simulink model "inverter_base"  (R2024a)
settings: Solver=VariableStepAuto  StartTime=0.0  StopTime=0.5  RelTol=1e-3
undefined symbols (not defined in the file): C_filter, L1, L2, R_damp, R_series1, R_series2
libraries: spsSeriesRLCBranchLib x5, spsIGBTDiodeLib x4, spsVoltageMeasurementLib x4, spsCurrentMeasurementLib x3, spsDCVoltageSourceLib x1, spspowerguiLib x1
settings Model: Creator=user  LastModifiedBy=user

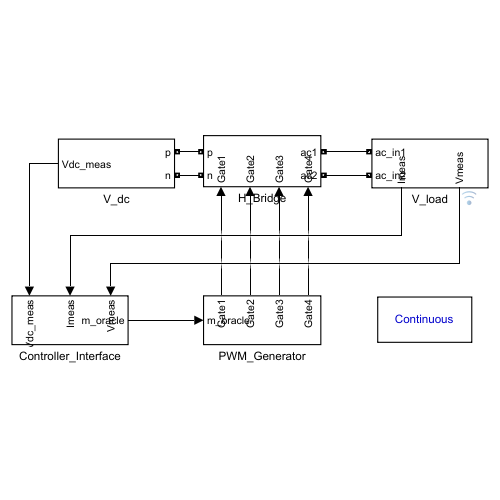
[thumbnail: Simulink's stored preview of the top-level diagram]
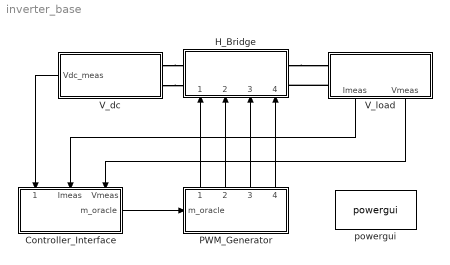
== system inverter_base ==
  Controller_Interface : Subsystem
      settings: PortSchema="{\"entries\":[{\"content\":{\"sides\":[{\"content\":{},\"type\":\"ConnectorPlacement.EquallySpacedRectSide\",\"uuid\":\"9a16cef6-3ad2-4b7e-9cb0-1cc099279abc\"},{\"content\":{\"connectorIds\":[\"Out1\"],\"side\":\"RIGHT\"},\"type\":\"ConnectorPlacement.EquallySpacedRectSide\",\"uuid\":\"1641ad69-610c-4562-8ab1-2b7cab01bb45\"},{\"content\":{\"connectorIds\":[\"In1\",\"In2\",\"In3\"],\"side\":\"TOP\"},\"type\":\"ConnectorPlacement.EquallySpacedRectSide\",\"uuid\":\"2c8d616f-a4b3-4b7e-a4a8-8a8252d3766c\"}]},\"type\":\"ConnectorPlacement.EquallySpacedConnector\",\"uuid\":\"2c20ff8a-19ba-4bf3-9a10-031d18a0fe42\"}],\"packageUris\":[\"http://schema.mathworks.com/mf0/Connector/R2020b\"],\"version\":\"1.0\"}"
  H_Bridge : Subsystem
      settings: PortSchema="{\"entries\":[{\"content\":{\"sides\":[{\"content\":{\"connectorIds\":[\"LConn1\",\"LConn2\"]},\"type\":\"ConnectorPlacement.EquallySpacedRectSide\",\"uuid\":\"86489d03-198d-4d40-a5a9-bb389f882c52\"},{\"content\":{\"connectorIds\":[\"RConn1\",\"RConn2\"],\"side\":\"RIGHT\"},\"type\":\"ConnectorPlacement.EquallySpacedRectSide\",\"uuid\":\"3ab0f84a-d55a-4cb1-90b5-b7bc956b0bff\"},{\"content\":{\"side\":\"TOP\"},\"type\":\"ConnectorPlacement.EquallySpacedRectSide\",\"uuid\":\"23383f72-5c44-4878-8c70-727696e5b54e\"},{\"content\":{\"connectorIds\":[\"In1\",\"In2\",\"In3\",\"In4\"],\"side\":\"BOTTOM\"},\"type\":\"ConnectorPlacement.EquallySpacedRectSide\",\"uuid\":\"2d41232e-3b94-4b8d-8bb1-4fff68b55e28\"}]},\"type\":\"ConnectorPlacement.EquallySpacedConnector\",\"uuid\":\"d39d40f2-549c-43a5-af7d-108fa7f92b85\"}],\"packageUris\":[\"http://schema.mathworks.com/mf0/Connector/R2020b\"],\"version\":\"1.0\"}"
  PWM_Generator : Subsystem
      settings: PortSchema="{\"entries\":[{\"content\":{\"sides\":[{\"content\":{\"connectorIds\":[\"In1\"]},\"type\":\"ConnectorPlacement.EquallySpacedRectSide\",\"uuid\":\"400e631f-5393-4580-84ff-cf0e7a5cd70f\"},{\"content\":{\"side\":\"RIGHT\"},\"type\":\"ConnectorPlacement.EquallySpacedRectSide\",\"uuid\":\"fe659c7d-79b6-4ef2-8759-c3fa799506d4\"},{\"content\":{\"connectorIds\":[\"Out1\",\"Out2\",\"Out3\",\"Out4\"],\"side\":\"TOP\"},\"type\":\"ConnectorPlacement.EquallySpacedRectSide\",\"uuid\":\"3e9a409d-18be-4b1d-9bb1-0d4655d86115\"}]},\"type\":\"ConnectorPlacement.EquallySpacedConnector\",\"uuid\":\"2db352b5-5690-44f0-aaa9-f258dc14ff92\"}],\"packageUris\":[\"http://schema.mathworks.com/mf0/Connector/R2020b\"],\"version\":\"1.0\"}"
  V_dc : Subsystem
      settings: PortSchema="{\"entries\":[{\"content\":{\"sides\":[{\"content\":{\"connectorIds\":[\"Out1\"]},\"type\":\"ConnectorPlacement.EquallySpacedRectSide\",\"uuid\":\"2cb68214-b015-46eb-8931-ac971d781749\"},{\"content\":{\"connectorIds\":[\"RConn1\",\"RConn2\"],\"side\":\"RIGHT\"},\"type\":\"ConnectorPlacement.EquallySpacedRectSide\",\"uuid\":\"9d50e4c1-4d5c-4242-a631-3bd3e824d3e8\"},{\"content\":{\"side\":\"TOP\"},\"type\":\"ConnectorPlacement.EquallySpacedRectSide\",\"uuid\":\"afad02bd-f500-4aa5-b819-b29c92a1000c\"},{\"content\":{\"side\":\"BOTTOM\"},\"type\":\"ConnectorPlacement.EquallySpacedRectSide\",\"uuid\":\"d1fcf53c-bcc4-4453-a05d-028d0bdae388\"}]},\"type\":\"ConnectorPlacement.EquallySpacedConnector\",\"uuid\":\"cb259193-6dd3-4248-8ce6-c0a2b09c3017\"}],\"packageUris\":[\"http://schema.mathworks.com/mf0/Connector/R2020b\"],\"version\":\"1.0\"}"
  V_load : Subsystem
      settings: PortSchema="{\"entries\":[{\"content\":{\"sides\":[{\"content\":{\"connectorIds\":[\"LConn1\",\"LConn2\"]},\"type\":\"ConnectorPlacement.EquallySpacedRectSide\",\"uuid\":\"e1621729-e0e3-4406-9722-79cabe3ad09b\"},{\"content\":{\"side\":\"RIGHT\"},\"type\":\"ConnectorPlacement.EquallySpacedRectSide\",\"uuid\":\"78182f87-e3d0-42da-9ed2-9ba8ffc9d138\"},{\"content\":{\"side\":\"TOP\"},\"type\":\"ConnectorPlacement.EquallySpacedRectSide\",\"uuid\":\"2eb99f15-710b-4356-9e1d-01d85ed72129\"},{\"content\":{\"connectorIds\":[\"Out1\",\"Out2\"],\"side\":\"BOTTOM\"},\"type\":\"ConnectorPlacement.EquallySpacedRectSide\",\"uuid\":\"a27496c2-30d5-461e-bcd5-c52dd3d0006a\"}]},\"type\":\"ConnectorPlacement.EquallySpacedConnector\",\"uuid\":\"2b7d626a-0ed9-442a-a508-e7f793cba935\"}],\"packageUris\":[\"http://schema.mathworks.com/mf0/Connector/R2020b\"],\"version\":\"1.0\"}"
  powergui : spspowerguiLib/powergui  Priority=1  SimulationMode=Continuous  SampleTime=50e-6  frequency=60  Iterations=50  frequencyindice=0  Pbase=100e6  ErrMax=1e-4  UnitsV=kV  UnitsW=MW  buscounter=0  FunctionMessages=off  echomessages=off  EnableUseOfTLC=off  CurrentSourceSwitches=off  DisableSnubberDevices=off  DisableRonSwitches=off  DisableVfSwitches=off  DisplayEquations=off  AutomaticDiscreteSolvers=off  SolverType=Tustin/Backward Euler (TBE)  Interpol=off  ExternalGateDelay=off  methode=off  Ts=100  x0status=blocks  SPID=on  SwTol=0  HookPort=off  NonlinearTolerance=1e-4  nMaxIteration=100  ContinueOnMaxIteration=off  RestoreLinks=warning  ResistiveCurrentMeasurement=off  Frange=[0:2:500]  Ylog=off  Xlog=on  ShowGrid=off  save=off  variable=ZData  structure=0  ZoomFFT=off  StartTime=0.0  cycles=1  DisplayStyle=1  fundamental=60  FreqAxis=off  MaxFrequency=1000  frequencyindicesteady=1  RmsSteady=1  display=off
  wires:
  V_load/2(Vmeas) -> Controller_Interface/3(Vmeas)
  V_dc/1(Vdc_meas) -> Controller_Interface/1(Vdc_meas)
  V_load/1(Imeas) -> Controller_Interface/2(Imeas)
  PWM_Generator/1(Gate1) -> H_Bridge/1(Gate1)
  PWM_Generator/2(Gate2) -> H_Bridge/2(Gate2)
  PWM_Generator/3(Gate3) -> H_Bridge/3(Gate3)
  PWM_Generator/4(Gate4) -> H_Bridge/4(Gate4)
  Controller_Interface/1(m_oracle) -> PWM_Generator/1(m_oracle)
  connections:
  V_dc/RConn1 -- H_Bridge/LConn1
  V_dc/RConn2 -- H_Bridge/LConn2
  H_Bridge/RConn1 -- V_load/LConn1
  V_load/LConn2 -- H_Bridge/RConn2

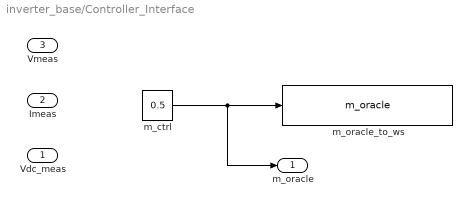
== system inverter_base/Controller_Interface ==
  Vdc_meas : Inport
  Imeas : Inport  Port=2
  Vmeas : Inport  Port=3
  m_ctrl : Constant  Value=0.5
  m_oracle_to_ws : ToWorkspace  VariableName=m_oracle  SaveFormat=Structure With Time  SampleTime=-1
  m_oracle : Outport
  wires:
  m_ctrl/1 -> m_oracle/1, m_oracle_to_ws/1

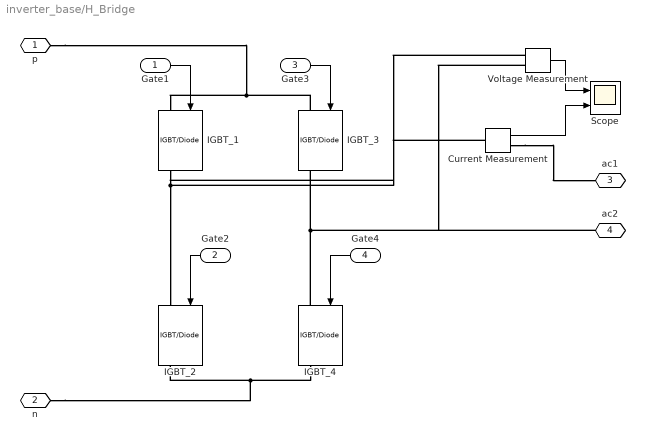
== system inverter_base/H_Bridge ==
  Gate1 : Inport
  Gate2 : Inport  Port=2
  Gate3 : Inport  Port=3
  Gate4 : Inport  Port=4
  Current Measurement : spsCurrentMeasurementLib/Current Measurement  PhasorSimulation=off  OutputType=Complex  PSBequivalent=0
  IGBT_{1..4} (4 alike) : spsIGBTDiodeLib/IGBT//Diode  Ron=1e-3  Rs=1e5  Cs=inf  Measurements=on
  Scope : Scope  NumInputPorts=2
  Voltage Measurement : spsVoltageMeasurementLib/Voltage Measurement  PhasorSimulation=off  OutputType=Complex  PSBequivalent=0
  p : PMIOPort  Side=Left
  n : PMIOPort  Port=2  Side=Left
  ac1 : PMIOPort  Port=3  Side=Right
  ac2 : PMIOPort  Port=4  Side=Right
  wires:
  Gate1/1 -> IGBT_1/1
  Gate3/1 -> IGBT_3/1
  Gate2/1 -> IGBT_2/1
  Gate4/1 -> IGBT_4/1
  Voltage Measurement/1 -> Scope/1
  Current Measurement/1 -> Scope/2
  connections:
  IGBT_4/RConn1 -- IGBT_2/RConn1 -- n/RConn1
  IGBT_3/LConn1 -- p/RConn1 -- IGBT_1/LConn1
  IGBT_1/RConn1 -- Current Measurement/LConn1 -- Voltage Measurement/LConn1 -- IGBT_2/LConn1
  IGBT_4/LConn1 -- Voltage Measurement/LConn2 -- ac2/RConn1 -- IGBT_3/RConn1
  Current Measurement/RConn1 -- ac1/RConn1

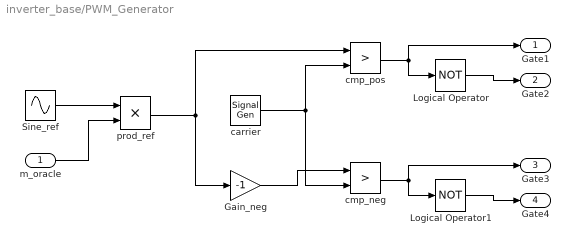
== system inverter_base/PWM_Generator ==
  m_oracle : Inport
  Gain_neg : Gain  Gain=-1
  Logical Operator : Logic  Operator=NOT  Inputs=1  AllPortsSameDT=off  OutDataTypeStr=boolean
  Logical Operator1 : Logic  Operator=NOT  Inputs=1  AllPortsSameDT=off  OutDataTypeStr=boolean
  Sine_ref : Sin  Frequency=2*pi*50  SampleTime=0
  carrier : SignalGenerator  WaveForm=sawtooth  Frequency=8000
  cmp_neg : RelationalOperator  Operator=>  OutDataTypeStr=boolean  RndMeth=Simplest  InputSameDT=off
  cmp_pos : RelationalOperator  Operator=>  OutDataTypeStr=boolean  RndMeth=Simplest  InputSameDT=off
  prod_ref : Product
  Gate1 : Outport
  Gate2 : Outport  Port=2
  Gate3 : Outport  Port=3
  Gate4 : Outport  Port=4
  wires:
  Sine_ref/1 -> prod_ref/1
  m_oracle/1 -> prod_ref/2
  prod_ref/1 -> cmp_pos/1, Gain_neg/1
  carrier/1 -> cmp_neg/2, cmp_pos/2
  Gain_neg/1 -> cmp_neg/1
  cmp_pos/1 -> Gate1/1, Logical Operator/1
  Logical Operator/1 -> Gate2/1
  cmp_neg/1 -> Gate3/1, Logical Operator1/1
  Logical Operator1/1 -> Gate4/1

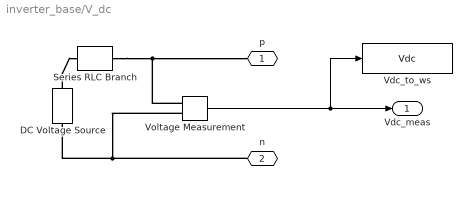
== system inverter_base/V_dc ==
  DC Voltage Source : spsDCVoltageSourceLib/DC Voltage Source  Amplitude=400  Measurements=Voltage
  Series RLC Branch : spsSeriesRLCBranchLib/Series RLC Branch  LConnTagsString=__new0  RConnTagsString=__new0  BranchType=R  Resistance=0.1  Inductance=1e-3  SetiL0=off  InitialCurrent=0  Capacitance=1e-6  Setx0=off  InitialVoltage=0  Measurements=None
  Vdc_to_ws : ToWorkspace  VariableName=Vdc  SaveFormat=Structure With Time  SampleTime=-1
  Voltage Measurement : spsVoltageMeasurementLib/Voltage Measurement  PhasorSimulation=off  OutputType=Complex  PSBequivalent=0
  p : PMIOPort  Side=Right
  n : PMIOPort  Port=2  Side=Right
  Vdc_meas : Outport
  wires:
  Voltage Measurement/1 -> Vdc_meas/1, Vdc_to_ws/1
  connections:
  DC Voltage Source/RConn1 -- Series RLC Branch/LConn1
  n/RConn1 -- DC Voltage Source/LConn1 -- Voltage Measurement/LConn2
  Series RLC Branch/RConn1 -- Voltage Measurement/LConn1 -- p/RConn1

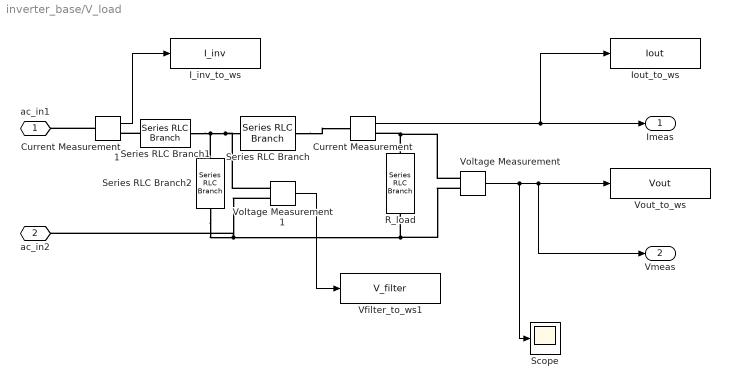
== system inverter_base/V_load ==
  Current Measurement : spsCurrentMeasurementLib/Current Measurement  PhasorSimulation=off  OutputType=Complex  PSBequivalent=0
  Current Measurement1 : spsCurrentMeasurementLib/Current Measurement  PhasorSimulation=off  OutputType=Complex  PSBequivalent=0
  I_inv_to_ws : ToWorkspace  VariableName=I_inv  SaveFormat=Structure With Time  SampleTime=-1
  Iout_to_ws : ToWorkspace  VariableName=Iout  SaveFormat=Structure With Time  SampleTime=-1
  R_load : spsSeriesRLCBranchLib/Series RLC Branch  LConnTagsString=__new0  RConnTagsString=__new0  BranchType=R  Resistance=10  Inductance=3e-3  SetiL0=on  InitialCurrent=0  Capacitance=1e-6  Setx0=off  InitialVoltage=0  Measurements=None
  Scope : Scope
  Series RLC Branch : spsSeriesRLCBranchLib/Series RLC Branch  LConnTagsString=__new0  RConnTagsString=__new0  BranchType=RL  Resistance=R_series2  Inductance=L2  SetiL0=off  InitialCurrent=0  Capacitance=1e-6  Setx0=off  InitialVoltage=0  Measurements=None
  Series RLC Branch1 : spsSeriesRLCBranchLib/Series RLC Branch  LConnTagsString=__new0  RConnTagsString=__new0  BranchType=RL  Resistance=R_series1  Inductance=L1  SetiL0=off  InitialCurrent=0  Capacitance=1e-6  Setx0=off  InitialVoltage=0  Measurements=None
  Series RLC Branch2 : spsSeriesRLCBranchLib/Series RLC Branch  LConnTagsString=__new0  RConnTagsString=__new0  BranchType=RC  Resistance=R_damp  Inductance=1e-3  SetiL0=off  InitialCurrent=0  Capacitance=C_filter  Setx0=off  InitialVoltage=0  Measurements=None
  Vfilter_to_ws1 : ToWorkspace  VariableName=V_filter  SaveFormat=Structure With Time  SampleTime=-1
  Voltage Measurement : spsVoltageMeasurementLib/Voltage Measurement  PhasorSimulation=off  OutputType=Complex  PSBequivalent=0
  Voltage Measurement1 : spsVoltageMeasurementLib/Voltage Measurement  PhasorSimulation=off  OutputType=Complex  PSBequivalent=0
  Vout_to_ws : ToWorkspace  VariableName=Vout  SaveFormat=Structure With Time  SampleTime=-1
  ac_in1 : PMIOPort  Side=Left
  ac_in2 : PMIOPort  Port=2  Side=Left
  Imeas : Outport
  Vmeas : Outport  Port=2
  wires:
  Voltage Measurement/1 -> Scope/1, Vmeas/1, Vout_to_ws/1
  Current Measurement/1 -> Iout_to_ws/1, Imeas/1
  Current Measurement1/1 -> I_inv_to_ws/1
  Voltage Measurement1/1 -> Vfilter_to_ws1/1
  connections:
  Current Measurement1/LConn1 -- ac_in1/RConn1
  Series RLC Branch2/RConn1 -- ac_in2/RConn1 -- Voltage Measurement1/LConn2 -- Voltage Measurement/LConn2 -- R_load/RConn1
  R_load/LConn1 -- Voltage Measurement/LConn1 -- Current Measurement/RConn1
  Series RLC Branch/RConn1 -- Current Measurement/LConn1
  Series RLC Branch1/LConn1 -- Current Measurement1/RConn1
  Series RLC Branch1/RConn1 -- Voltage Measurement1/LConn1 -- Series RLC Branch/LConn1 -- Series RLC Branch2/LConn1
